simulink model "MPC_control"  (R2018a)
settings: Solver=FixedStepAuto  StartTime=0  StopTime=Tend  FixedStep=0.001  RelTol=5e-3
model workspace (MAT data in the model file):
  A_mu = 10
  B_reff = 8.386
  Cz = 7766.25
  DCT_Param : struct (value not decoded)
  D_reff = 0.25826
  Downshift_Speeds = [9.5625 12.9375 16.3125 19.6875 23.0625 26.4375 29.8125 33.1875 36.5625 39.9375 43.3125 46.6875 ... (28 elements, 4x7)]
  Pedal_Positions = [0.1 0.4 0.5 0.9]
  SUS : struct (value not decoded)
  Upshift_Speeds = [12.9375 16.3125 19.6875 33 26.4375 29.8125 33.1875 52.5 39.9375 43.3125 46.6875 77.25 ... (28 elements, 4x7)]
  VEH : struct (value not decoded)
  V_o = 16.7
  V_xlow = 1
  WH : struct (value not decoded)
  a = 1.4
  alpha_max = 1.5
  alpha_min = -1.5
  b = 1.8
  c_zo = 209651
  epsilon = 0.1
  h = 0.134
  path : struct (value not decoded)
  pio = 220000
  q_Fcx = 0
  q_Fz2 = 15.4
  q_Fzy = 0
  q_reo = 0.9974
  q_sx1 = -0.007764
  q_sx10 = 0.2824
  q_sx11 = 5.349
  q_sx12 = 0
  q_sx13 = 0
  q_sx14 = 0
  q_sx2 = 1.1915
  q_sx3 = 0.013948
  q_sx4 = 4.912
  q_sx5 = 1.02
  q_sx6 = 22.83
  q_sx7 = 0.7104
  q_sx8 = -0.023393
  q_sx9 = 0.6581
  q_sy1 = 0.00702
  q_sy2 = 0
  q_sy3 = 0.001515
  q_sy4 = 8.514e-05
  q_sy5 = 0
  q_sy6 = 0
  q_sy7 = 0.9008
  q_sy8 = -0.4089
  q_v1 = 0.0007742
  q_v2 = 0.04667
  r_Bx1 = 12.531
  r_Bx2 = 9.532
  r_Bx3 = 0
  r_By1 = 10.615
  r_By2 = 7.705
  r_By3 = 3.433e-06
  r_By4 = 0
  r_Cx1 = 1.019
  r_Cy1 = 1.0585
  r_Ex1 = -0.4487
  r_Ex2 = -0.4726
  r_Ey1 = 0.3132
  r_Ey2 = 7.63e-06
  r_Hx1 = 0.0002374
  r_Hy1 = 0.011646
  r_Hy2 = 7.63e-06
  r_Vy1 = 0.05654
  r_Vy2 = 7.63e-06
  r_Vy3 = 0
  r_Vy4 = 99.9
  r_Vy5 = 2
  r_Vy6 = 15.814
  r_o = 0.3135
  vehWidth = 2
  w = 1
symbols that are objects in the model workspace (value not decoded): VEH
undefined symbols (not defined in the file): Cok_1, Cok_2, Cok_3, Cok_4, Cok_5, Cok_6, Cok_7, Cok_8, Cok_9, Cout_1, Cout_2, Cout_3, Cout_4, Cout_5, Cout_6, Cout_7, Cout_8, Cout_9, DiscIntNeverNeededParam, Dout_1, Dout_2, Dout_3, Dout_4, Dout_5, Dout_6, Dout_7, Dout_8, Dout_9, F_1, F_2, F_3, F_4, F_5, F_6, F_7, F_8, F_9, Gd_1, Gd_2, Gd_3, Gd_4, Gd_5, Gd_6, Gd_7, Gd_8, Gd_9, Gok_1, Gok_2, Gok_3, Gok_4, Gok_5, Gok_6, Gok_7, Gok_8, Gok_9, Gsys_2, Gsys_9, Hd_1, Hd_2, Hd_3 ... (+70)
libraries: robotalgslib x10, simulink x5, sim3dlib x2, autolibutils x1, vehdynlibviscommon x1
(part 2 of 5)

== system MPC_control/Visualization/3D Engine ==
  note: 1) Add Subsystem or Model blocks as valid variant choices.
      | 2) You cannot connect blocks at this level. At simulation, connectivity is automatically
      | determined, based on the active variant and port name matching.
  VehFdbk : Inport
  3D Engine : Subsystem  VariantControl=1
  3D Engine Disabled : Subsystem  VariantControl=0

== system MPC_control/Visualization/Acceleration Cmd ==

== system MPC_control/Visualization/Brake Cmd ==

== system MPC_control/Visualization/Engine Tach [rpm] ==

== system MPC_control/Visualization/Handwheel Angle [deg] ==

== system MPC_control/Visualization/Lateral Acceleration [g] ==

== system MPC_control/Visualization/Speed [mph] ==

== system MPC_control/Visualization/Vehicle XY Plotter ==
  VehFdbk : Inport
  Bus Selector1 : BusSelector  OutputSignals=Body.phi,Body.theta,Body.psi  OutputAsBus=on
  Bus Selector2 : BusSelector  OutputSignals=Driveline.WhlAng  OutputAsBus=on
  Bus Selector3 : BusSelector  OutputSignals=Body.X,Body.Y,Body.Z  OutputAsBus=on
  Bus Selector4 : BusSelector  OutputSignals=Body.Xdot,Body.Ydot  OutputAsBus=on
  Bus to Vector{,1..3} (4 alike) : BusToVector
  Ground : Ground
  Rate Transition{1..2,5..6} (4 alike) : RateTransition  OutPortSampleTime=pltDT
  Vector Concatenate : Concatenate
  Vehicle XY Plotter : vehdynlibviscommon/Vehicle XY Plotter  bufferSize=bufferSize  w=w  a=a  b=b
  wires:
  Bus to Vector2/1 -> Rate Transition1/1  "InertCGDisp"
  Rate Transition5/1 -> Vehicle XY Plotter/1
  Bus Selector4/1 -> Bus to Vector1/1
  Rate Transition1/1 -> Vehicle XY Plotter/2
  Rate Transition6/1 -> Vehicle XY Plotter/3
  Vector Concatenate/1 -> Rate Transition6/1  "InertCGVel"
  Bus Selector1/1 -> Bus to Vector2/1
  Bus to Vector/1 -> Rate Transition5/1  "InertCGDisp"
  Bus Selector3/1 -> Bus to Vector/1
  Bus to Vector1/1 -> Vector Concatenate/1
  Ground/1 -> Vector Concatenate/2
  Bus to Vector3/1 -> Rate Transition2/1
  Bus Selector2/1 -> Bus to Vector3/1
  VehFdbk/1 -> Bus Selector1/1, Bus Selector2/1, Bus Selector4/1, Bus Selector3/1
  Rate Transition2/1 -> Vehicle XY Plotter/4

== system MPC_control/observer_of_plant/Subsystem_1 ==
  select_MPC : Inport
  select_overlap : Inport  Port=2
  select_overlap2 : Inport  Port=3
  initial : Inport  Port=4
  r(k) : Inport  Port=5
  r(k-1) : Inport  Port=6
  U(k) : Inport  Port=7
  U(k-1) : Inport  Port=8
  Y(k) : Inport  Port=9
  Demux2 : Demux  Outputs=3
  From Workspace : FromWorkspace  VariableName=flag_mod1  SampleTime=0
  gate1 : MATLAB Function  TreatAsAtomicUnit=on
  observer_of_simulator_1 : Subsystem
  simulator_1 : Subsystem
  xhat : Outport
  sye : Outport  Port=2
  ope : Outport  Port=3
  wires:
  simulator_1/2(U_overlap) -> observer_of_simulator_1/2(U_overlap)
  observer_of_simulator_1/1(xhat) -> xhat/1, simulator_1/9(xhat)
  simulator_1/1(Y_overlap) -> observer_of_simulator_1/5(Y_overlap)
  Demux2/2 -> simulator_1/4(Initial Velocities)
  Demux2/3 -> simulator_1/5(Initial HeadingAngles)
  Demux2/1 -> simulator_1/3(Initial position)
  Y(k)/1 -> observer_of_simulator_1/6(Y)
  initial/1 -> Demux2/1
  select_overlap/1 -> gate1/2(select_overlap)
  select_MPC/1 -> gate1/1(select_MPC)
  select_overlap2/1 -> gate1/3(select_overlap2)
  gate1/1(state_MPC) -> simulator_1/1(select_MPC)
  gate1/2(state_overlap) -> observer_of_simulator_1/1(select_overlap), simulator_1/2(select_overlap)
  r(k)/1 -> simulator_1/6(r(k))
  r(k-1)/1 -> observer_of_simulator_1/7(r(k-1)), simulator_1/7(r(k-1))
  U(k)/1 -> observer_of_simulator_1/3(U)
  U(k-1)/1 -> observer_of_simulator_1/4(U(k-1)), simulator_1/8(U(k-1))
  From Workspace/1 -> simulator_1/Enable
  observer_of_simulator_1/2(sye) -> sye/1
  observer_of_simulator_1/3(ope) -> ope/1

== system MPC_control/observer_of_plant/Subsystem_2 ==
  select_MPC : Inport
  select_overlap : Inport  Port=2
  select_overlap2 : Inport  Port=3
  initial : Inport  Port=4
  r(k) : Inport  Port=5
  r(k-1) : Inport  Port=6
  U(k) : Inport  Port=7
  U(k-1) : Inport  Port=8
  Y(k) : Inport  Port=9
  Demux2 : Demux  Outputs=3
  From Workspace1 : FromWorkspace  VariableName=flag_mod2  SampleTime=0
  gate2 : MATLAB Function  TreatAsAtomicUnit=on
  observer_of_simulator_2 : Subsystem
  simulator_2 : Subsystem
  xhat : Outport
  sye : Outport  Port=2
  ope : Outport  Port=3
  wires:
  simulator_2/2(U_overlap) -> observer_of_simulator_2/2(U_overlap)
  observer_of_simulator_2/1(xhat) -> xhat/1, simulator_2/9(xhat)
  simulator_2/1(Y_overlap) -> observer_of_simulator_2/5(Y_overlap)
  Demux2/2 -> simulator_2/4(Initial Velocities)
  Demux2/3 -> simulator_2/5(Initial HeadingAngles)
  Demux2/1 -> simulator_2/3(Initial position)
  Y(k)/1 -> observer_of_simulator_2/6(Y)
  initial/1 -> Demux2/1
  observer_of_simulator_2/2(sye) -> sye/1
  observer_of_simulator_2/3(ope) -> ope/1
  gate2/1(state_MPC) -> simulator_2/1(select_MPC)
  gate2/2(state_overlap) -> simulator_2/2(select_overlap), observer_of_simulator_2/1(select_overlap)
  select_MPC/1 -> gate2/1(select_MPC)
  select_overlap/1 -> gate2/2(select_overlap)
  select_overlap2/1 -> gate2/3(select_overlap2)
  From Workspace1/1 -> simulator_2/Enable
  r(k)/1 -> simulator_2/6(r(k))
  r(k-1)/1 -> observer_of_simulator_2/7(r(k-1)), simulator_2/7(r(k-1))
  U(k-1)/1 -> observer_of_simulator_2/4(U(k-1)), simulator_2/8(U(k-1))
  U(k)/1 -> observer_of_simulator_2/3(U)

== system MPC_control/observer_of_plant/Subsystem_3 ==
  select_MPC : Inport
  select_overlap : Inport  Port=2
  select_overlap2 : Inport  Port=3
  initial : Inport  Port=4
  r(k) : Inport  Port=5
  r(k-1) : Inport  Port=6
  U(k) : Inport  Port=7
  U(k-1) : Inport  Port=8
  Y(k) : Inport  Port=9
  Demux2 : Demux  Outputs=3
  From Workspace2 : FromWorkspace  VariableName=flag_mod3  SampleTime=0
  gate3 : MATLAB Function  TreatAsAtomicUnit=on
  observer_of_simulator_3 : Subsystem
  simulator_3 : Subsystem
  xhat : Outport
  sye : Outport  Port=2
  ope : Outport  Port=3
  wires:
  simulator_3/2(U_overlap) -> observer_of_simulator_3/2(U_overlap)
  simulator_3/1(Y_overlap) -> observer_of_simulator_3/5(Y_overlap)
  Demux2/2 -> simulator_3/4(Initial Velocities)
  Demux2/3 -> simulator_3/5(Initial HeadingAngles)
  Demux2/1 -> simulator_3/3(Initial position)
  Y(k)/1 -> observer_of_simulator_3/6(Y)
  initial/1 -> Demux2/1
  gate3/1(state_MPC) -> simulator_3/1(select_MPC)
  gate3/2(state_overlap) -> simulator_3/2(select_overlap), observer_of_simulator_3/1(select_overlap)
  select_MPC/1 -> gate3/1(select_MPC)
  select_overlap/1 -> gate3/2(select_overlap)
  select_overlap2/1 -> gate3/3(select_overlap2)
  r(k)/1 -> simulator_3/6(r(k))
  r(k-1)/1 -> observer_of_simulator_3/7(r(k-1)), simulator_3/7(r(k-1))
  U(k)/1 -> observer_of_simulator_3/3(U)
  U(k-1)/1 -> observer_of_simulator_3/4(U(k-1)), simulator_3/8(U(k-1))
  observer_of_simulator_3/1(xhat) -> xhat/1, simulator_3/9(xhat)
  observer_of_simulator_3/2(sye) -> sye/1
  observer_of_simulator_3/3(ope) -> ope/1
  From Workspace2/1 -> simulator_3/Enable

== system MPC_control/observer_of_plant/Subsystem_4 ==
  select_MPC : Inport
  select_overlap : Inport  Port=2
  select_overlap2 : Inport  Port=3
  initial : Inport  Port=4
  r(k) : Inport  Port=5
  r(k-1) : Inport  Port=6
  U(k) : Inport  Port=7
  U(k-1) : Inport  Port=8
  Y(k) : Inport  Port=9
  Demux2 : Demux  Outputs=3
  From Workspace3 : FromWorkspace  VariableName=flag_mod4  SampleTime=0
  gate4 : MATLAB Function  TreatAsAtomicUnit=on
  observer_of_simulator_4 : Subsystem
  simulator_4 : Subsystem
  xhat : Outport
  sye : Outport  Port=2
  ope : Outport  Port=3
  wires:
  simulator_4/2(U_overlap) -> observer_of_simulator_4/2(U_overlap)
  simulator_4/1(Y_overlap) -> observer_of_simulator_4/5(Y_overlap)
  Demux2/2 -> simulator_4/4(Initial Velocities)
  Demux2/3 -> simulator_4/5(Initial HeadingAngles)
  Demux2/1 -> simulator_4/3(Initial position)
  Y(k)/1 -> observer_of_simulator_4/6(Y)
  initial/1 -> Demux2/1
  U(k)/1 -> observer_of_simulator_4/3(U)
  gate4/1(state_MPC) -> simulator_4/1(select_MPC)
  gate4/2(state_overlap) -> simulator_4/2(select_overlap), observer_of_simulator_4/1(select_overlap)
  select_MPC/1 -> gate4/1(select_MPC)
  select_overlap/1 -> gate4/2(select_overlap)
  select_overlap2/1 -> gate4/3(select_overlap2)
  r(k)/1 -> simulator_4/6(r(k))
  r(k-1)/1 -> simulator_4/7(r(k-1)), observer_of_simulator_4/7(r(k-1))
  U(k-1)/1 -> simulator_4/8(U(k-1)), observer_of_simulator_4/4(U(k-1))
  From Workspace3/1 -> simulator_4/Enable
  observer_of_simulator_4/1(xhat) -> simulator_4/9(xhat), xhat/1
  observer_of_simulator_4/2(sye) -> sye/1
  observer_of_simulator_4/3(ope) -> ope/1

== system MPC_control/observer_of_plant/Subsystem_5 ==
  select_MPC : Inport
  select_overlap : Inport  Port=2
  select_overlap2 : Inport  Port=3
  initial : Inport  Port=4
  r(k) : Inport  Port=5
  r(k-1) : Inport  Port=6
  U(k) : Inport  Port=7
  U(k-1) : Inport  Port=8
  Y(k) : Inport  Port=9
  Demux2 : Demux  Outputs=3
  From Workspace4 : FromWorkspace  VariableName=flag_mod5  SampleTime=0
  gate5 : MATLAB Function  TreatAsAtomicUnit=on
  observer_of_simulator_5 : Subsystem
  simulator_5 : Subsystem
  xhat : Outport
  sye : Outport  Port=2
  ope : Outport  Port=3
  wires:
  simulator_5/2(U_overlap) -> observer_of_simulator_5/2(U_overlap)
  simulator_5/1(Y_overlap) -> observer_of_simulator_5/5(Y_overlap)
  Demux2/2 -> simulator_5/4(Initial Velocities)
  Demux2/3 -> simulator_5/5(Initial HeadingAngles)
  Demux2/1 -> simulator_5/3(Initial position)
  Y(k)/1 -> observer_of_simulator_5/6(Y)
  initial/1 -> Demux2/1
  gate5/1(state_MPC) -> simulator_5/1(select_MPC)
  gate5/2(state_overlap) -> observer_of_simulator_5/1(select_overlap), simulator_5/2(select_overlap)
  select_MPC/1 -> gate5/1(select_MPC)
  select_overlap/1 -> gate5/2(select_overlap)
  select_overlap2/1 -> gate5/3(select_overlap2)
  r(k)/1 -> simulator_5/6(r(k))
  U(k-1)/1 -> observer_of_simulator_5/4(U(k-1)), simulator_5/8(U(k-1))
  From Workspace4/1 -> simulator_5/Enable
  observer_of_simulator_5/1(xhat) -> simulator_5/9(xhat), xhat/1
  observer_of_simulator_5/2(sye) -> sye/1
  observer_of_simulator_5/3(ope) -> ope/1
  r(k-1)/1 -> observer_of_simulator_5/7(r(k-1)), simulator_5/7(r(k-1))
  U(k)/1 -> observer_of_simulator_5/3(U)

== system MPC_control/observer_of_plant/Subsystem_6 ==
  select_MPC : Inport
  select_overlap : Inport  Port=2
  select_overlap1 : Inport  Port=3
  initial : Inport  Port=4
  r(k) : Inport  Port=5
  r(k-1) : Inport  Port=6
  U(k) : Inport  Port=7
  U(k-1) : Inport  Port=8
  Y(k) : Inport  Port=9
  Demux2 : Demux  Outputs=3
  From Workspace5 : FromWorkspace  VariableName=flag_mod6  SampleTime=0
  gate6 : MATLAB Function  TreatAsAtomicUnit=on
  observer_of_simulator_6 : Subsystem
  simulator_6 : Subsystem
  xhat : Outport
  sye : Outport  Port=2
  ope : Outport  Port=3
  wires:
  simulator_6/2(U_overlap) -> observer_of_simulator_6/2(U_overlap)
  simulator_6/1(Y_overlap) -> observer_of_simulator_6/5(Y_overlap)
  Demux2/2 -> simulator_6/4(Initial Velocities)
  Demux2/3 -> simulator_6/5(Initial HeadingAngles)
  Demux2/1 -> simulator_6/3(Initial position)
  Y(k)/1 -> observer_of_simulator_6/6(Y)
  initial/1 -> Demux2/1
  gate6/1(state_MPC) -> simulator_6/1(select_MPC)
  gate6/2(state_overlap) -> observer_of_simulator_6/1(select_overlap), simulator_6/2(select_overlap)
  select_MPC/1 -> gate6/1(select_MPC)
  select_overlap/1 -> gate6/2(select_overlap)
  select_overlap1/1 -> gate6/3(select_overlap2)
  r(k)/1 -> simulator_6/6(r(k))
  U(k)/1 -> observer_of_simulator_6/3(U)
  U(k-1)/1 -> observer_of_simulator_6/4(U(k-1)), simulator_6/8(U(k-1))
  observer_of_simulator_6/1(xhat) -> xhat/1, simulator_6/9(xhat)
  observer_of_simulator_6/2(sye) -> sye/1
  observer_of_simulator_6/3(ope) -> ope/1
  From Workspace5/1 -> simulator_6/Enable
  r(k-1)/1 -> observer_of_simulator_6/7(r(k-1)), simulator_6/7(r(k-1))

== system MPC_control/observer_of_plant/Subsystem_7 ==
  select_MPC : Inport
  select_overlap : Inport  Port=2
  select_overlap2 : Inport  Port=3
  initial : Inport  Port=4
  r(k) : Inport  Port=5
  r(k-1) : Inport  Port=6
  U(k) : Inport  Port=7
  U(k-1) : Inport  Port=8
  Y(k) : Inport  Port=9
  Demux2 : Demux  Outputs=3
  From Workspace6 : FromWorkspace  VariableName=flag_mod7  SampleTime=0
  gate7 : MATLAB Function  TreatAsAtomicUnit=on
  observer_of_simulator_7 : Subsystem
  simulator_7 : Subsystem
  xhat : Outport
  sye : Outport  Port=2
  ope : Outport  Port=3
  wires:
  simulator_7/2(U_overlap) -> observer_of_simulator_7/2(U_overlap)
  observer_of_simulator_7/1(xhat) -> xhat/1, simulator_7/9(xhat)
  simulator_7/1(Y_overlap) -> observer_of_simulator_7/5(Y_overlap)
  Demux2/2 -> simulator_7/4(Initial Velocities)
  Demux2/3 -> simulator_7/5(Initial HeadingAngles)
  Demux2/1 -> simulator_7/3(Initial position)
  Y(k)/1 -> observer_of_simulator_7/6(Y)
  initial/1 -> Demux2/1
  gate7/1(state_MPC) -> simulator_7/1(select_MPC)
  gate7/2(state_overlap) -> simulator_7/2(select_overlap), observer_of_simulator_7/1(select_overlap)
  select_MPC/1 -> gate7/1(select_MPC)
  select_overlap/1 -> gate7/2(select_overlap)
  select_overlap2/1 -> gate7/3(select_overlap2)
  r(k)/1 -> simulator_7/6(r(k))
  r(k-1)/1 -> observer_of_simulator_7/7(r(k-1)), simulator_7/7(r(k-1))
  U(k)/1 -> observer_of_simulator_7/3(U)
  U(k-1)/1 -> observer_of_simulator_7/4(U(k-1)), simulator_7/8(U(k-1))
  observer_of_simulator_7/2(sye) -> sye/1
  observer_of_simulator_7/3(ope) -> ope/1
  From Workspace6/1 -> simulator_7/Enable

== system MPC_control/observer_of_plant/Subsystem_8 ==
  select_MPC : Inport
  select_overlap : Inport  Port=2
  select_overlap2 : Inport  Port=3
  initial : Inport  Port=4
  r(k) : Inport  Port=5
  r(k-1) : Inport  Port=6
  U(k) : Inport  Port=7
  U(k-1) : Inport  Port=8
  Y(k) : Inport  Port=9
  Demux2 : Demux  Outputs=3
  From Workspace7 : FromWorkspace  VariableName=flag_mod8  SampleTime=0
  gate8 : MATLAB Function  TreatAsAtomicUnit=on
  observer_of_simulator_8 : Subsystem
  simulator_8 : Subsystem
  xhat : Outport
  sye : Outport  Port=2
  ope : Outport  Port=3
  wires:
  simulator_8/2(U_overlap) -> observer_of_simulator_8/2(U_overlap)
  simulator_8/1(Y_overlap) -> observer_of_simulator_8/5(Y_overlap)
  Demux2/2 -> simulator_8/4(Initial Velocities)
  Demux2/3 -> simulator_8/5(Initial HeadingAngles)
  Demux2/1 -> simulator_8/3(Initial position)
  Y(k)/1 -> observer_of_simulator_8/6(Y)
  initial/1 -> Demux2/1
  gate8/1(state_MPC) -> simulator_8/1(select_MPC)
  gate8/2(state_overlap) -> observer_of_simulator_8/1(select_overlap), simulator_8/2(select_overlap)
  select_MPC/1 -> gate8/1(select_MPC)
  select_overlap/1 -> gate8/2(select_overlap)
  select_overlap2/1 -> gate8/3(select_overlap2)
  r(k)/1 -> simulator_8/6(r(k))
  r(k-1)/1 -> observer_of_simulator_8/7(r(k-1)), simulator_8/7(r(k-1))
  U(k)/1 -> observer_of_simulator_8/3(U)
  U(k-1)/1 -> observer_of_simulator_8/4(U(k-1)), simulator_8/8(U(k-1))
  observer_of_simulator_8/1(xhat) -> xhat/1, simulator_8/9(xhat)
  observer_of_simulator_8/2(sye) -> sye/1
  observer_of_simulator_8/3(ope) -> ope/1
  From Workspace7/1 -> simulator_8/Enable

== system MPC_control/observer_of_plant/Subsystem_9 ==
  select_MPC : Inport
  select_overlap : Inport  Port=2
  select_overlap2 : Inport  Port=3
  initial : Inport  Port=4
  r(k) : Inport  Port=5
  r(k-1) : Inport  Port=6
  U(k) : Inport  Port=7
  U(k-1) : Inport  Port=8
  Y(k) : Inport  Port=9
  Demux2 : Demux  Outputs=3
  From Workspace8 : FromWorkspace  VariableName=flag_mod9  SampleTime=0
  gate9 : MATLAB Function  TreatAsAtomicUnit=on
  observer_of_simulator_9 : Subsystem
  simulator_9 : Subsystem
  xhat : Outport
  sye : Outport  Port=2
  ope : Outport  Port=3
  wires:
  simulator_9/2(U_overlap) -> observer_of_simulator_9/2(U_overlap)
  observer_of_simulator_9/1(xhat) -> xhat/1, simulator_9/9(xhat)
  simulator_9/1(Y_overlap) -> observer_of_simulator_9/5(Y_overlap)
  Demux2/2 -> simulator_9/4(Initial Velocities)
  Demux2/3 -> simulator_9/5(Initial HeadingAngles)
  Demux2/1 -> simulator_9/3(Initial position)
  Y(k)/1 -> observer_of_simulator_9/6(Y)
  initial/1 -> Demux2/1
  observer_of_simulator_9/2(sye) -> sye/1
  observer_of_simulator_9/3(ope) -> ope/1
  gate9/1(state_MPC) -> simulator_9/1(select_MPC)
  gate9/2(state_overlap) -> simulator_9/2(select_overlap), observer_of_simulator_9/1(select_overlap)
  select_MPC/1 -> gate9/1(select_MPC)
  select_overlap/1 -> gate9/2(select_overlap)
  select_overlap2/1 -> gate9/3(select_overlap2)
  From Workspace8/1 -> simulator_9/Enable
  r(k)/1 -> simulator_9/6(r(k))
  r(k-1)/1 -> simulator_9/7(r(k-1)), observer_of_simulator_9/7(r(k-1))
  U(k-1)/1 -> simulator_9/8(U(k-1)), observer_of_simulator_9/4(U(k-1))
  U(k)/1 -> observer_of_simulator_9/3(U)

== system MPC_control/Controllers/Brake Controller/Brake Pressure Control ==
  note: 1) Add Subsystem or Model blocks as valid variant choices.
      | 2) You cannot connect blocks at this level. At simulation, connectivity is automatically
      | determined, based on the active variant and port name matching.
  Pref : Inport
  xdot : Inport  Port=2
  <Kappa> : Inport  Port=3
  Bang Bang ABS : Subsystem  VariantControl=1
  Open Loop : Subsystem  VariantControl=0
  PCmd : Outport

== system MPC_control/Controllers/Transmission Controller/TCM ==
  AccCmd : Inport
  EngSpd : Inport  Port=2
  VehSpdFdbk : Inport  Port=3
  function : TriggerPort  TriggerType=function-call  VariantControl=Variant
  Neutral Select : Subsystem
  Prop Shaft Speed LPF : DiscreteTransferFcn  Numerator=[0.000000000000000 0.009950166250832 ]  Denominator=[1.000000000000000 -0.990049833749168 ]  mask(DiscretizedDiscreteTransferFcn){}
      mask init:
      | %zoh
  TCM Shift Controller : Stateflow chart  TreatAsAtomicUnit=on
  prop speed to vehicle speed : Gain  Gain=0.45
  Gear Select : Outport
  wires:
  VehSpdFdbk/1 -> Prop Shaft Speed LPF/1
  TCM Shift Controller/1(GearState) -> Gear Select/1  "GearCmd"
  AccCmd/1 -> Neutral Select/1(AccCmd), TCM Shift Controller/2(pedal)  "AccCmd"
  Neutral Select/1(Neutral Select) -> TCM Shift Controller/3(Neutral)
  EngSpd/1 -> Neutral Select/2(EngSpd)
  prop speed to vehicle speed/1 -> TCM Shift Controller/1(speed)
  Prop Shaft Speed LPF/1 -> prop speed to vehicle speed/1

== system MPC_control/Visualization/3D Engine/3D Engine ==
  VehFdbk : Inport
  3D Body Offset : Constant  Value=single(0.0112)  OutDataTypeStr=single
  Add1 : Sum  Inputs=-+
  Add3 : Sum  Inputs=-+-
  Bus Selector : BusSelector  OutputSignals=Body.X,Body.Y,Body.Z,Body.phi,Body.theta,Body.psi
  Bus Selector2 : BusSelector  OutputSignals=Wheels.zAxle,Wheels.omega,Driveline.WhlAng
  Bus Selector3 : BusSelector  OutputSignals=Body.ZHP
  Constant1 : Constant  Value=zeros(4,1)  OutDataTypeStr=single
  Constant2 : Constant  Value=0  OutDataTypeStr=single
  Constant8 : Constant  Value=h
  Data Type Conversion{1,4..10,12} (9 alike) : DataTypeConversion  OutDataTypeStr=single
  Demux{,1..3} (4 alike) : Demux
  Integrator : Integrator  WrapState=on  WrappedStateUpperValue=2*pi  WrappedStateLowerValue=0  ZeroCross=off
  Part Rotation Concatenation : Subsystem
  Part Translation Concatenation : Subsystem
  Rate Transition : RateTransition  OutPortSampleTime=dt3D
  Scale : Subsystem
  Simulation 3D Engine 1 : sim3dlib/Simulation 3D Config  Priority=1  ProjectFormat=Executable  ProjectName=VehicleSimulation.exe  SceneDesc=Straight road  OpVisEn=off  Ts=dt3D
      settings: AttributesFormatString=Priority: %<Priority>
  Unary Minus : UnaryMinus
  Vehicle Actor Transform Set : sim3dlib/Simulation 3D Actor Transform Set  ActorTag=SimulinkVehicle1  ActorType=Passenger vehicle  PassVehMesh=Muscle car  VehColor=Red  NumberOfParts=5  CustNumOfParts=3  Translation=[0 0 1; 0 0 0; 0 0 0; 0 0 0; 0 0 0]  Rotation=[0 0 0; 0 0 0; 0 0 0; 0 0 0; 0 0 0]  Scale=[1 1 1; 1 1 1; 1 1 1; 1 1 1; 1 1 1]  Ts=dt3D
  wires:
  Unary Minus/1 -> Integrator/1
  Bus Selector3/1 -> Add3/2  "<ZHP>"
  Add3/1 -> Data Type Conversion12/1
  Bus Selector2/1 -> Add3/3  "<zAxle>"
  Constant8/1 -> Add3/1
  Rate Transition/1 -> Bus Selector/1, Bus Selector3/1, Bus Selector2/1
  Scale/1(ScaleOut) -> Vehicle Actor Transform Set/3
  Demux/4 -> Part Rotation Concatenation/7(WheelRearRight Ptich)
  Demux/3 -> Part Rotation Concatenation/6(WheelRearLeft Pitch)
  Demux/2 -> Part Rotation Concatenation/5(WheelFrontRight Pitch)
  Demux/1 -> Part Rotation Concatenation/4(WheelFrontLeft Pitch)
  Constant1/1 -> Demux2/1
  Bus Selector/4 -> Data Type Conversion7/1  "<phi>"
  Data Type Conversion6/1 -> Add1/1
  Part Rotation Concatenation/1(ConcatOut) -> Vehicle Actor Transform Set/2
  Part Translation Concatenation/1(ConcatOut) -> Vehicle Actor Transform Set/1
  Data Type Conversion12/1 -> Demux3/1
  Demux3/4 -> Part Translation Concatenation/15(WheelRearRightZ)
  Demux3/3 -> Part Translation Concatenation/14(WheelRearLeftZ)
  Demux3/1 -> Part Translation Concatenation/12(WheelFrontLeftZ)
  Demux3/2 -> Part Translation Concatenation/13(WheelFrontRightZ)
  VehFdbk/1 -> Rate Transition/1
  Add1/1 -> Part Translation Concatenation/3(BodyZ)
  3D Body Offset/1 -> Add1/2
  Demux1/4 -> Part Rotation Concatenation/15(WheelRearRight Yaw)
  Demux1/3 -> Part Rotation Concatenation/14(WheelRearLeft Yaw)
  Demux2/1 -> Part Rotation Concatenation/8(WheelFrontLeft Roll)
  Demux2/2 -> Part Rotation Concatenation/9(WheelFrontRight Roll)
  Demux2/3 -> Part Rotation Concatenation/10(WheelRearLeft Roll)
  Demux2/4 -> Part Rotation Concatenation/11(WheelRearRight Roll)
  Bus Selector2/3 -> Data Type Conversion9/1  "<WhlAng>"
  Bus Selector2/2 -> Unary Minus/1  "<omega>"
  Data Type Conversion9/1 -> Demux1/1
  Demux1/1 -> Part Rotation Concatenation/12(WheelFrontLeft Yaw)
  Demux1/2 -> Part Rotation Concatenation/13(WheelFrontRight Yaw)
  Integrator/1 -> Data Type Conversion1/1
  Data Type Conversion1/1 -> Demux/1
  Data Type Conversion8/1 -> Part Rotation Concatenation/2(Body Ptich)
  Data Type Conversion5/1 -> Part Translation Concatenation/2(BodyY)
  Data Type Conversion10/1 -> Part Rotation Concatenation/3(Body Yaw)
  Constant2/1 -> Part Translation Concatenation/5(WheelFrontRightX), Part Translation Concatenation/6(WheelRearLeftX), Part Translation Concatenation/7(WheelRearRightX), Part Translation Concatenation/8(WheelFrontLeftY), Part Translation Concatenation/9(WheelFrontRightY), Part Translation Concatenation/10(WheelRearLeftY), Part Translation Concatenation/11(WheelRearRightY), Part Translation Concatenation/4(WheelFrontLeftX)
  Data Type Conversion4/1 -> Part Translation Concatenation/1(BodyX)
  Data Type Conversion7/1 -> Part Rotation Concatenation/1(Body Roll)
  Bus Selector/1 -> Data Type Conversion4/1  "<X>"
  Bus Selector/2 -> Data Type Conversion5/1  "<Y>"
  Bus Selector/3 -> Data Type Conversion6/1  "<Z>"
  Bus Selector/6 -> Data Type Conversion10/1  "<psi>"
  Bus Selector/5 -> Data Type Conversion8/1  "<theta>"

== system MPC_control/Visualization/3D Engine/3D Engine Disabled ==
  VehFdbk : Inport
  Terminator : Terminator
  wires:
  VehFdbk/1 -> Terminator/1

== system MPC_control/observer_of_plant/Subsystem_1/observer_of_simulator_1 ==
  select_overlap : Inport
  U_overlap : Inport  Port=2
  U : Inport  Port=3
  U(k-1) : Inport  Port=4
  Y_overlap : Inport  Port=5
  Y : Inport  Port=6
  r(k-1) : Inport  Port=7
  Cok_1 : Gain  Gain=Cok_1  Multiplication=Matrix(K*u) (u vector)
  Cok_1* : Gain  Gain=Cok_1  Multiplication=Matrix(K*u) (u vector)
  Delay : Delay  DelayLength=1  InitialConditionSource=Input port  InitialCondition=0  ExternalReset=Rising  SampleTime=Ts
      settings: InputPortMap=u0,r5,p4
  Delay1 : Delay  DelayLength=1  InitialConditionSource=Input port  InitialCondition=0  ExternalReset=Rising  SampleTime=Ts
      settings: InputPortMap=u0,r5,p4
  Gd_1 : Gain  Gain=Gd_1  Multiplication=Matrix(K*u) (u vector)
  Gok_1 : Gain  Gain=Gok_1  Multiplication=Matrix(K*u) (u vector)
  Hd_1 : Gain  Gain=Hd_1  Multiplication=Matrix(K*u) (u vector)
  Hok_1 : Gain  Gain=Hok_1  Multiplication=Matrix(K*u) (u vector)
  Ld_1 : Gain  Gain=Ld_1  Multiplication=Matrix(K*u) (u vector)
  Ld_1* : Gain  Gain=Ld_1  Multiplication=Matrix(K*u) (u vector)
  Sum : Sum  Inputs=|-+
  Sum1 : Sum
  Sum2 : Sum  Inputs=|-+
  Sum4 : Sum  Inputs=+++
  Switch1 : Switch  Threshold=1
  Switch2 : Switch  Threshold=1
  xhat : Outport
  sye : Outport  Port=2
  ope : Outport  Port=3
  wires:
  Hd_1/1 -> Sum4/2
  Ld_1/1 -> Sum4/1
  Delay1/1 -> Hok_1/1, Hd_1/1
  U_overlap/1 -> Switch2/1
  Gd_1/1 -> Sum4/3
  Y/1 -> Sum/2, Sum2/2, Switch1/3
  U/1 -> Switch2/3
  Sum4/1 -> xhat/1, Cok_1/1, Delay/1  "xhat"
  Delay/1 -> Gok_1/1, Gd_1/1
  Y_overlap/1 -> Switch1/1
  U(k-1)/1 -> Delay1/3
  select_overlap/1 -> Delay/2, Delay1/2, Switch2/2, Switch1/2
  r(k-1)/1 -> Ld_1*/1
  Switch1/1 -> Ld_1/1
  Switch2/1 -> Delay1/1
  Ld_1*/1 -> Delay/3
  Cok_1/1 -> Sum/1
  Hok_1/1 -> Sum1/2
  Gok_1/1 -> Sum1/1
  Sum1/1 -> Cok_1*/1
  Cok_1*/1 -> Sum2/1
  Sum2/1 -> sye/1
  Sum/1 -> ope/1

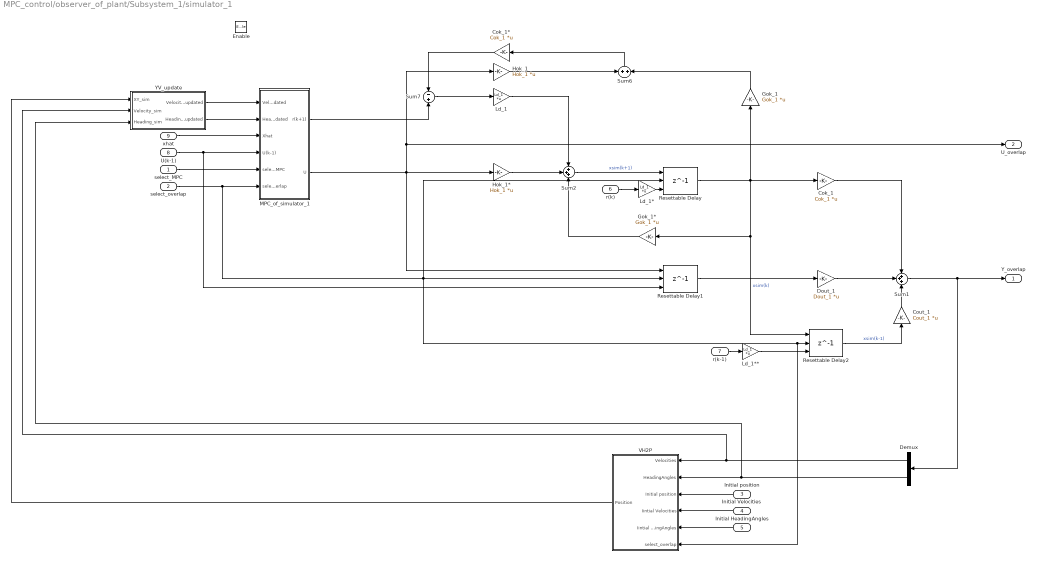
== system MPC_control/observer_of_plant/Subsystem_1/simulator_1 ==
  select_MPC : Inport
  select_overlap : Inport  Port=2
  Initial position : Inport  Port=3
  Initial Velocities : Inport  Port=4
  Initial HeadingAngles : Inport  Port=5
  r(k) : Inport  Port=6
  r(k-1) : Inport  Port=7
  U(k-1) : Inport  Port=8
  xhat : Inport  Port=9
  Enable : EnablePort
  Cok_1 : Gain  Gain=Cok_1  Multiplication=Matrix(K*u) (u vector)
  Cok_1* : Gain  Gain=Cok_1  Multiplication=Matrix(K*u) (u vector)
  Cout_1 : Gain  Gain=Cout_1  Multiplication=Matrix(K*u) (u vector)
  Demux : Demux  Outputs=2
  Dout_1 : Gain  Gain=Dout_1  Multiplication=Matrix(K*u) (u vector)
  Gok_1 : Gain  Gain=Gok_1  Multiplication=Matrix(K*u) (u vector)
  Gok_1* : Gain  Gain=Gok_1  Multiplication=Matrix(K*u) (u vector)
  Hok_1 : Gain  Gain=Hok_1  Multiplication=Matrix(K*u) (u vector)
  Hok_1* : Gain  Gain=Hok_1  Multiplication=Matrix(K*u) (u vector)
  Ld_1 : Gain  Gain=Ld_1  Multiplication=Matrix(K*u) (u vector)
  Ld_1* : Gain  Gain=Ld_1  Multiplication=Matrix(K*u) (u vector)
  Ld_1** : Gain  Gain=Ld_1  Multiplication=Matrix(K*u) (u vector)
  MPC_of_simulator_1 : Subsystem
  Resettable Delay : Delay  DelayLength=1  InitialConditionSource=Input port  ExternalReset=Rising  SampleTime=Ts
      settings: InputPortMap=u0,r5,p4
  Resettable Delay1 : Delay  DelayLength=1  InitialConditionSource=Input port  ExternalReset=Rising  SampleTime=Ts
      settings: InputPortMap=u0,r5,p4
  Resettable Delay2 : Delay  DelayLength=1  InitialConditionSource=Input port  ExternalReset=Rising  SampleTime=Ts
      settings: InputPortMap=u0,r5,p4
  Sum1 : Sum  Inputs=+++
  Sum2 : Sum  Inputs=+++
  Sum6 : Sum
  Sum7 : Sum  Inputs=-+
  VH2P : Subsystem
  YV_update : Subsystem  TreatAsAtomicUnit=on
  Y_overlap : Outport
  U_overlap : Outport  Port=2
  wires:
  Initial position/1 -> VH2P/3(Initial position)
  Sum2/1 -> Resettable Delay/1  "xsim(k+1)"
  Demux/2 -> VH2P/2(HeadingAngles), YV_update/3(Heading_sim)
  Ld_1/1 -> Sum2/1
  Sum7/1 -> Ld_1/1
  Cout_1/1 -> Sum1/3
  MPC_of_simulator_1/2(U) -> Resettable Delay1/1, Hok_1*/1, U_overlap/1, Hok_1/1
  Hok_1*/1 -> Sum2/2
  Gok_1*/1 -> Sum2/3
  Resettable Delay2/1 -> Cout_1/1  "xsim(k-1)"
  VH2P/1(Position) -> YV_update/1(XY_sim)
  Demux/1 -> YV_update/2(Velocity_sim), VH2P/1(Velocities)
  Resettable Delay/1 -> Gok_1*/1, Resettable Delay2/1, Gok_1/1, Cok_1/1  "xsim(k)"
  Hok_1/1 -> Sum6/1
  Sum1/1 -> Y_overlap/1, Demux/1
  Sum6/1 -> Cok_1*/1
  Dout_1/1 -> Sum1/2
  Resettable Delay1/1 -> Dout_1/1
  Cok_1/1 -> Sum1/1
  YV_update/2(Heading_updated) -> MPC_of_simulator_1/2(Heading_updated)
  YV_update/1(Velocity_updated) -> MPC_of_simulator_1/1(Velocity_updated)
  r(k)/1 -> Ld_1*/1
  Ld_1*/1 -> Resettable Delay/3
  U(k-1)/1 -> MPC_of_simulator_1/4(U(k-1)), Resettable Delay1/3
  r(k-1)/1 -> Ld_1**/1
  Ld_1**/1 -> Resettable Delay2/3
  Initial Velocities/1 -> VH2P/4(Iintial Velocities)
  Initial HeadingAngles/1 -> VH2P/5(Iintial HeadingAngles)
  select_overlap/1 -> MPC_of_simulator_1/6(select_overlap), Resettable Delay/2, VH2P/6(select_overlap), Resettable Delay2/2, Resettable Delay1/2
  Gok_1/1 -> Sum6/2
  Cok_1*/1 -> Sum7/1
  select_MPC/1 -> MPC_of_simulator_1/5(select_MPC)
  MPC_of_simulator_1/1(r(k+1)) -> Sum7/2
  xhat/1 -> MPC_of_simulator_1/3(Xhat)

== system MPC_control/observer_of_plant/Subsystem_2/observer_of_simulator_2 ==
  select_overlap : Inport
  U_overlap : Inport  Port=2
  U : Inport  Port=3
  U(k-1) : Inport  Port=4
  Y_overlap : Inport  Port=5
  Y : Inport  Port=6
  r(k-1) : Inport  Port=7
  Cok_2 : Gain  Gain=Cok_2  Multiplication=Matrix(K*u) (u vector)
  Cok_2* : Gain  Gain=Cok_2  Multiplication=Matrix(K*u) (u vector)
  Delay : Delay  DelayLength=1  InitialConditionSource=Input port  InitialCondition=0  ExternalReset=Rising  SampleTime=Ts
      settings: InputPortMap=u0,r5,p4
  Delay1 : Delay  DelayLength=1  InitialConditionSource=Input port  InitialCondition=0  ExternalReset=Rising  SampleTime=Ts
      settings: InputPortMap=u0,r5,p4
  Gd_2 : Gain  Gain=Gd_2  Multiplication=Matrix(K*u) (u vector)
  Gok_2 : Gain  Gain=Gok_2  Multiplication=Matrix(K*u) (u vector)
  Hd_2 : Gain  Gain=Hd_2  Multiplication=Matrix(K*u) (u vector)
  Hok_2 : Gain  Gain=Hok_2  Multiplication=Matrix(K*u) (u vector)
  Ld_2 : Gain  Gain=Ld_2  Multiplication=Matrix(K*u) (u vector)
  Ld_2* : Gain  Gain=Ld_2  Multiplication=Matrix(K*u) (u vector)
  Sum : Sum  Inputs=|-+
  Sum1 : Sum
  Sum2 : Sum  Inputs=|-+
  Sum4 : Sum  Inputs=+++
  Switch1 : Switch  Threshold=1
  Switch2 : Switch  Threshold=1
  xhat : Outport
  sye : Outport  Port=2
  ope : Outport  Port=3
  wires:
  Hd_2/1 -> Sum4/2
  Ld_2/1 -> Sum4/1
  U_overlap/1 -> Switch2/1
  Gd_2/1 -> Sum4/3
  U/1 -> Switch2/3
  Y_overlap/1 -> Switch1/1
  U(k-1)/1 -> Delay1/3
  select_overlap/1 -> Delay/2, Delay1/2, Switch2/2, Switch1/2
  r(k-1)/1 -> Ld_2*/1
  Switch1/1 -> Ld_2/1
  Switch2/1 -> Delay1/1
  Ld_2*/1 -> Delay/3
  Delay/1 -> Gok_2/1, Gd_2/1
  Sum2/1 -> sye/1
  Sum/1 -> ope/1
  Cok_2/1 -> Sum/1
  Hok_2/1 -> Sum1/2
  Delay1/1 -> Hok_2/1, Hd_2/1
  Gok_2/1 -> Sum1/1
  Y/1 -> Sum/2, Sum2/2, Switch1/3
  Cok_2*/1 -> Sum2/1
  Sum1/1 -> Cok_2*/1
  Sum4/1 -> xhat/1, Cok_2/1, Delay/1  "xhat"

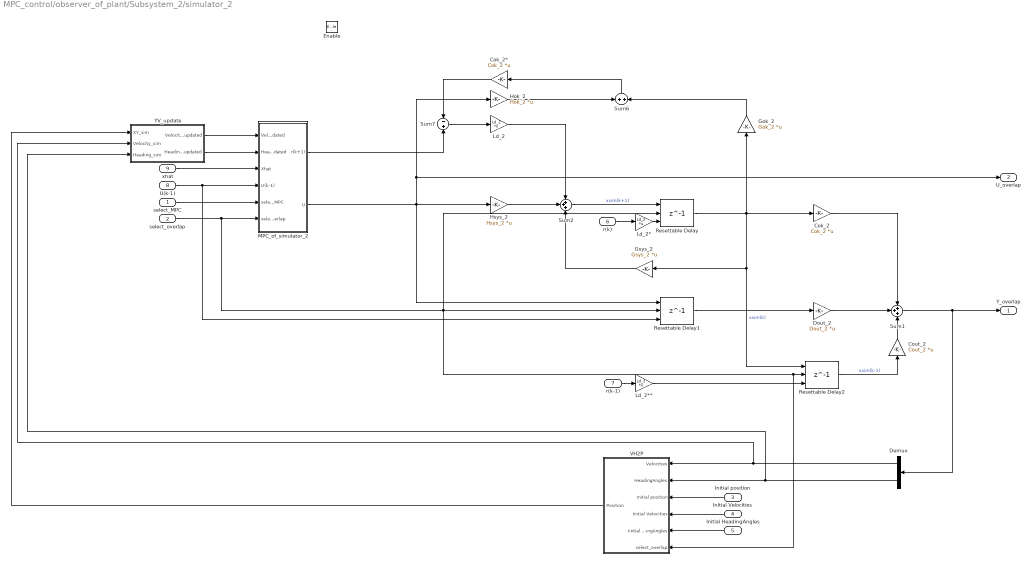
== system MPC_control/observer_of_plant/Subsystem_2/simulator_2 ==
  select_MPC : Inport
  select_overlap : Inport  Port=2
  Initial position : Inport  Port=3
  Initial Velocities : Inport  Port=4
  Initial HeadingAngles : Inport  Port=5
  r(k) : Inport  Port=6
  r(k-1) : Inport  Port=7
  U(k-1) : Inport  Port=8
  xhat : Inport  Port=9
  Enable : EnablePort
  Cok_2 : Gain  Gain=Cok_2  Multiplication=Matrix(K*u) (u vector)
  Cok_2* : Gain  Gain=Cok_2  Multiplication=Matrix(K*u) (u vector)
  Cout_2 : Gain  Gain=Cout_2  Multiplication=Matrix(K*u) (u vector)
  Demux : Demux  Outputs=2
  Dout_2 : Gain  Gain=Dout_2  Multiplication=Matrix(K*u) (u vector)
  Gok_2 : Gain  Gain=Gok_2  Multiplication=Matrix(K*u) (u vector)
  Gsys_2 : Gain  Gain=Gsys_2  Multiplication=Matrix(K*u) (u vector)
  Hok_2 : Gain  Gain=Hok_2  Multiplication=Matrix(K*u) (u vector)
  Hsys_2 : Gain  Gain=Hsys_2  Multiplication=Matrix(K*u) (u vector)
  Ld_2 : Gain  Gain=Ld_2  Multiplication=Matrix(K*u) (u vector)
  Ld_2* : Gain  Gain=Ld_2  Multiplication=Matrix(K*u) (u vector)
  Ld_2** : Gain  Gain=Ld_2  Multiplication=Matrix(K*u) (u vector)
  MPC_of_simulator_2 : Subsystem
  Resettable Delay : Delay  DelayLength=1  InitialConditionSource=Input port  ExternalReset=Rising  SampleTime=Ts
      settings: InputPortMap=u0,r5,p4
  Resettable Delay1 : Delay  DelayLength=1  InitialConditionSource=Input port  ExternalReset=Rising  SampleTime=Ts
      settings: InputPortMap=u0,r5,p4
  Resettable Delay2 : Delay  DelayLength=1  InitialConditionSource=Input port  ExternalReset=Rising  SampleTime=Ts
      settings: InputPortMap=u0,r5,p4
  Sum1 : Sum  Inputs=+++
  Sum2 : Sum  Inputs=+++
  Sum6 : Sum
  Sum7 : Sum  Inputs=-+
  VH2P : Subsystem
  YV_update : Subsystem  TreatAsAtomicUnit=on
  Y_overlap : Outport
  U_overlap : Outport  Port=2
  wires:
  Initial position/1 -> VH2P/3(Initial position)
  Sum2/1 -> Resettable Delay/1  "xsim(k+1)"
  Demux/2 -> VH2P/2(HeadingAngles), YV_update/3(Heading_sim)
  Ld_2/1 -> Sum2/1
  Sum7/1 -> Ld_2/1
  Cout_2/1 -> Sum1/3
  MPC_of_simulator_2/2(U) -> Hok_2/1, U_overlap/1, Resettable Delay1/1, Hsys_2/1
  Hsys_2/1 -> Sum2/2
  Gsys_2/1 -> Sum2/3
  Resettable Delay2/1 -> Cout_2/1  "xsim(k-1)"
  VH2P/1(Position) -> YV_update/1(XY_sim)
  Demux/1 -> YV_update/2(Velocity_sim), VH2P/1(Velocities)
  Resettable Delay/1 -> Gsys_2/1, Resettable Delay2/1, Gok_2/1, Cok_2/1  "xsim(k)"
  Hok_2/1 -> Sum6/1
  Sum6/1 -> Cok_2*/1
  Dout_2/1 -> Sum1/2
  Resettable Delay1/1 -> Dout_2/1
  Cok_2/1 -> Sum1/1
  YV_update/2(Heading_updated) -> MPC_of_simulator_2/2(Heading_updated)
  xhat/1 -> MPC_of_simulator_2/3(Xhat)
  YV_update/1(Velocity_updated) -> MPC_of_simulator_2/1(Velocity_updated)
  r(k)/1 -> Ld_2*/1
  Ld_2*/1 -> Resettable Delay/3
  U(k-1)/1 -> MPC_of_simulator_2/4(U(k-1)), Resettable Delay1/3
  r(k-1)/1 -> Ld_2**/1
  Ld_2**/1 -> Resettable Delay2/3
  Initial Velocities/1 -> VH2P/4(Iintial Velocities)
  Initial HeadingAngles/1 -> VH2P/5(Iintial HeadingAngles)
  select_overlap/1 -> MPC_of_simulator_2/6(select_overlap), Resettable Delay/2, VH2P/6(select_overlap), Resettable Delay2/2, Resettable Delay1/2
  Gok_2/1 -> Sum6/2
  Cok_2*/1 -> Sum7/1
  select_MPC/1 -> MPC_of_simulator_2/5(select_MPC)
  Sum1/1 -> Demux/1, Y_overlap/1
  MPC_of_simulator_2/1(r(k+1)) -> Sum7/2

== system MPC_control/observer_of_plant/Subsystem_3/observer_of_simulator_3 ==
  select_overlap : Inport
  U_overlap : Inport  Port=2
  U : Inport  Port=3
  U(k-1) : Inport  Port=4
  Y_overlap : Inport  Port=5
  Y : Inport  Port=6
  r(k-1) : Inport  Port=7
  Cok_3 : Gain  Gain=Cok_3  Multiplication=Matrix(K*u) (u vector)
  Cok_3* : Gain  Gain=Cok_3  Multiplication=Matrix(K*u) (u vector)
  Delay : Delay  DelayLength=1  InitialConditionSource=Input port  InitialCondition=0  ExternalReset=Rising  SampleTime=Ts
      settings: InputPortMap=u0,r5,p4
  Delay1 : Delay  DelayLength=1  InitialConditionSource=Input port  InitialCondition=0  ExternalReset=Rising  SampleTime=Ts
      settings: InputPortMap=u0,r5,p4
  Gd_3 : Gain  Gain=Gd_3  Multiplication=Matrix(K*u) (u vector)
  Gok_3 : Gain  Gain=Gok_3  Multiplication=Matrix(K*u) (u vector)
  Hd_3 : Gain  Gain=Hd_3  Multiplication=Matrix(K*u) (u vector)
  Hok_3 : Gain  Gain=Hok_3  Multiplication=Matrix(K*u) (u vector)
  Ld_3 : Gain  Gain=Ld_3  Multiplication=Matrix(K*u) (u vector)
  Ld_3* : Gain  Gain=Ld_3  Multiplication=Matrix(K*u) (u vector)
  Sum : Sum  Inputs=|-+
  Sum1 : Sum
  Sum2 : Sum  Inputs=|-+
  Sum4 : Sum  Inputs=+++
  Switch1 : Switch  Threshold=1
  Switch2 : Switch  Threshold=1
  xhat : Outport
  sye : Outport  Port=2
  ope : Outport  Port=3
  wires:
  Hd_3/1 -> Sum4/2
  Ld_3/1 -> Sum4/1
  U_overlap/1 -> Switch2/1
  Gd_3/1 -> Sum4/3
  U/1 -> Switch2/3
  Y_overlap/1 -> Switch1/1
  U(k-1)/1 -> Delay1/3
  select_overlap/1 -> Delay/2, Delay1/2, Switch2/2, Switch1/2
  r(k-1)/1 -> Ld_3*/1
  Switch1/1 -> Ld_3/1
  Switch2/1 -> Delay1/1
  Ld_3*/1 -> Delay/3
  Delay/1 -> Gok_3/1, Gd_3/1
  Sum2/1 -> sye/1
  Sum/1 -> ope/1
  Cok_3/1 -> Sum/1
  Hok_3/1 -> Sum1/2
  Delay1/1 -> Hok_3/1, Hd_3/1
  Gok_3/1 -> Sum1/1
  Y/1 -> Sum/2, Sum2/2, Switch1/3
  Cok_3*/1 -> Sum2/1
  Sum1/1 -> Cok_3*/1
  Sum4/1 -> xhat/1, Cok_3/1, Delay/1  "xhat"

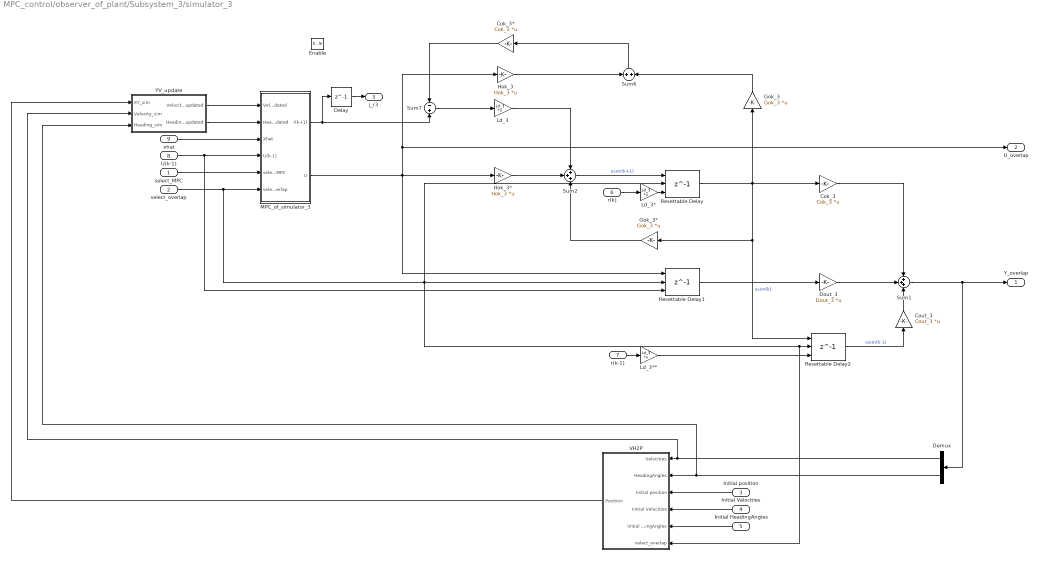
== system MPC_control/observer_of_plant/Subsystem_3/simulator_3 ==
  select_MPC : Inport
  select_overlap : Inport  Port=2
  Initial position : Inport  Port=3
  Initial Velocities : Inport  Port=4
  Initial HeadingAngles : Inport  Port=5
  r(k) : Inport  Port=6
  r(k-1) : Inport  Port=7
  U(k-1) : Inport  Port=8
  xhat : Inport  Port=9
  Enable : EnablePort
  Cok_3 : Gain  Gain=Cok_3  Multiplication=Matrix(K*u) (u vector)
  Cok_3* : Gain  Gain=Cok_3  Multiplication=Matrix(K*u) (u vector)
  Cout_3 : Gain  Gain=Cout_3  Multiplication=Matrix(K*u) (u vector)
  Delay : Delay  DelayLength=1  SampleTime=Ts
  Demux : Demux  Outputs=2
  Dout_3 : Gain  Gain=Dout_3  Multiplication=Matrix(K*u) (u vector)
  Gok_3 : Gain  Gain=Gok_3  Multiplication=Matrix(K*u) (u vector)
  Gok_3* : Gain  Gain=Gok_3  Multiplication=Matrix(K*u) (u vector)
  Hok_3 : Gain  Gain=Hok_3  Multiplication=Matrix(K*u) (u vector)
  Hok_3* : Gain  Gain=Hok_3  Multiplication=Matrix(K*u) (u vector)
  Ld_3 : Gain  Gain=Ld_3  Multiplication=Matrix(K*u) (u vector)
  Ld_3* : Gain  Gain=Ld_3  Multiplication=Matrix(K*u) (u vector)
  Ld_3** : Gain  Gain=Ld_3  Multiplication=Matrix(K*u) (u vector)
  MPC_of_simulator_3 : Subsystem
  Resettable Delay : Delay  DelayLength=1  InitialConditionSource=Input port  ExternalReset=Rising  SampleTime=Ts
      settings: InputPortMap=u0,r5,p4
  Resettable Delay1 : Delay  DelayLength=1  InitialConditionSource=Input port  ExternalReset=Rising  SampleTime=Ts
      settings: InputPortMap=u0,r5,p4
  Resettable Delay2 : Delay  DelayLength=1  InitialConditionSource=Input port  ExternalReset=Rising  SampleTime=Ts
      settings: InputPortMap=u0,r5,p4
  Sum1 : Sum  Inputs=+++
  Sum2 : Sum  Inputs=+++
  Sum6 : Sum
  Sum7 : Sum  Inputs=-+
  VH2P : Subsystem
  YV_update : Subsystem  TreatAsAtomicUnit=on
  Y_overlap : Outport
  U_overlap : Outport  Port=2
  j_r3 : Outport  Port=3
  wires:
  Sum2/1 -> Resettable Delay/1  "xsim(k+1)"
  Demux/2 -> VH2P/2(HeadingAngles), YV_update/3(Heading_sim)
  Ld_3/1 -> Sum2/1
  Sum7/1 -> Ld_3/1
  Cout_3/1 -> Sum1/3
  MPC_of_simulator_3/2(U) -> Resettable Delay1/1, Hok_3*/1, U_overlap/1, Hok_3/1
  Hok_3*/1 -> Sum2/2
  Gok_3*/1 -> Sum2/3
  Resettable Delay2/1 -> Cout_3/1  "xsim(k-1)"
  VH2P/1(Position) -> YV_update/1(XY_sim)
  Demux/1 -> YV_update/2(Velocity_sim), VH2P/1(Velocities)
  Resettable Delay/1 -> Gok_3*/1, Resettable Delay2/1, Gok_3/1, Cok_3/1  "xsim(k)"
  Hok_3/1 -> Sum6/1
  Sum6/1 -> Cok_3*/1
  Dout_3/1 -> Sum1/2
  Resettable Delay1/1 -> Dout_3/1
  Cok_3/1 -> Sum1/1
  YV_update/2(Heading_updated) -> MPC_of_simulator_3/2(Heading_updated)
  YV_update/1(Velocity_updated) -> MPC_of_simulator_3/1(Velocity_updated)
  r(k)/1 -> Ld_3*/1
  Ld_3*/1 -> Resettable Delay/3
  U(k-1)/1 -> MPC_of_simulator_3/4(U(k-1)), Resettable Delay1/3
  r(k-1)/1 -> Ld_3**/1
  Ld_3**/1 -> Resettable Delay2/3
  select_overlap/1 -> MPC_of_simulator_3/6(select_overlap), Resettable Delay/2, VH2P/6(select_overlap), Resettable Delay2/2, Resettable Delay1/2
  Gok_3/1 -> Sum6/2
  Cok_3*/1 -> Sum7/1
  select_MPC/1 -> MPC_of_simulator_3/5(select_MPC)
  Sum1/1 -> Demux/1, Y_overlap/1
  Delay/1 -> j_r3/1
  MPC_of_simulator_3/1(r(k+1)) -> Delay/1, Sum7/2
  Initial position/1 -> VH2P/3(Initial position)
  Initial Velocities/1 -> VH2P/4(Iintial Velocities)
  Initial HeadingAngles/1 -> VH2P/5(Iintial HeadingAngles)
  xhat/1 -> MPC_of_simulator_3/3(Xhat)

== system MPC_control/observer_of_plant/Subsystem_4/observer_of_simulator_4 ==
  select_overlap : Inport
  U_overlap : Inport  Port=2
  U : Inport  Port=3
  U(k-1) : Inport  Port=4
  Y_overlap : Inport  Port=5
  Y : Inport  Port=6
  r(k-1) : Inport  Port=7
  Cok_4 : Gain  Gain=Cok_4  Multiplication=Matrix(K*u) (u vector)
  Cok_4* : Gain  Gain=Cok_4  Multiplication=Matrix(K*u) (u vector)
  Delay : Delay  DelayLength=1  InitialConditionSource=Input port  InitialCondition=0  ExternalReset=Rising  SampleTime=Ts
      settings: InputPortMap=u0,r5,p4
  Delay1 : Delay  DelayLength=1  InitialConditionSource=Input port  InitialCondition=0  ExternalReset=Rising  SampleTime=Ts
      settings: InputPortMap=u0,r5,p4
  Gd_4 : Gain  Gain=Gd_4  Multiplication=Matrix(K*u) (u vector)
  Gok_4 : Gain  Gain=Gok_4  Multiplication=Matrix(K*u) (u vector)
  Hd_4 : Gain  Gain=Hd_4  Multiplication=Matrix(K*u) (u vector)
  Hok_4 : Gain  Gain=Hok_4  Multiplication=Matrix(K*u) (u vector)
  Ld_4 : Gain  Gain=Ld_4  Multiplication=Matrix(K*u) (u vector)
  Ld_4* : Gain  Gain=Ld_4  Multiplication=Matrix(K*u) (u vector)
  Sum : Sum  Inputs=|-+
  Sum1 : Sum
  Sum2 : Sum  Inputs=|-+
  Sum4 : Sum  Inputs=+++
  Switch1 : Switch  Threshold=1
  Switch2 : Switch  Threshold=1
  xhat : Outport
  sye : Outport  Port=2
  ope : Outport  Port=3
  wires:
  Hd_4/1 -> Sum4/2
  Ld_4/1 -> Sum4/1
  U_overlap/1 -> Switch2/1
  Gd_4/1 -> Sum4/3
  U/1 -> Switch2/3
  Y_overlap/1 -> Switch1/1
  U(k-1)/1 -> Delay1/3
  select_overlap/1 -> Delay/2, Delay1/2, Switch2/2, Switch1/2
  r(k-1)/1 -> Ld_4*/1
  Switch1/1 -> Ld_4/1
  Switch2/1 -> Delay1/1
  Ld_4*/1 -> Delay/3
  Delay/1 -> Gok_4/1, Gd_4/1
  Sum2/1 -> sye/1
  Sum/1 -> ope/1
  Cok_4/1 -> Sum/1
  Hok_4/1 -> Sum1/2
  Delay1/1 -> Hok_4/1, Hd_4/1
  Gok_4/1 -> Sum1/1
  Y/1 -> Sum/2, Sum2/2, Switch1/3
  Cok_4*/1 -> Sum2/1
  Sum1/1 -> Cok_4*/1
  Sum4/1 -> xhat/1, Cok_4/1, Delay/1  "xhat"

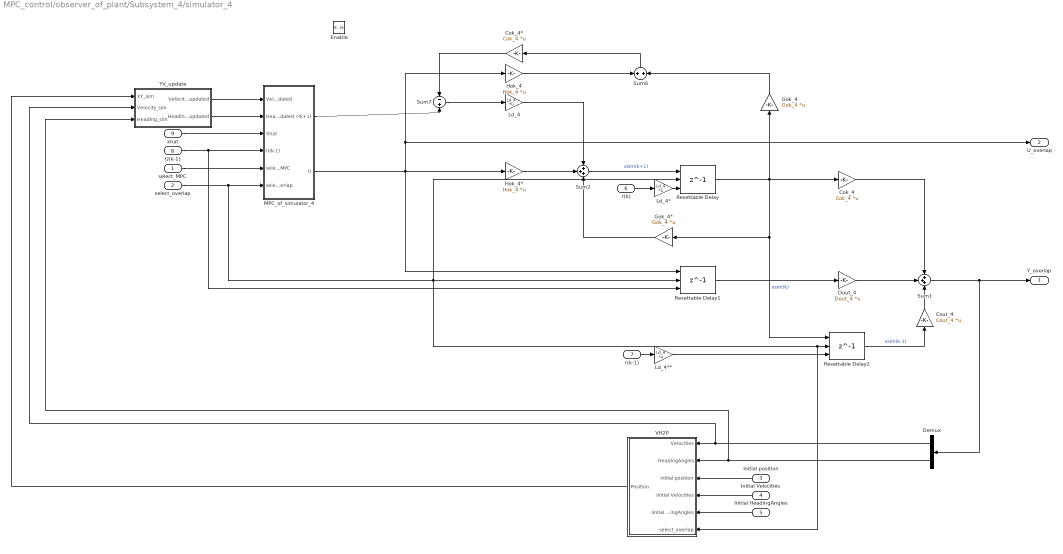
== system MPC_control/observer_of_plant/Subsystem_4/simulator_4 ==
  select_MPC : Inport
  select_overlap : Inport  Port=2
  Initial position : Inport  Port=3
  Initial Velocities : Inport  Port=4
  Initial HeadingAngles : Inport  Port=5
  r(k) : Inport  Port=6
  r(k-1) : Inport  Port=7
  U(k-1) : Inport  Port=8
  xhat : Inport  Port=9
  Enable : EnablePort
  Cok_4 : Gain  Gain=Cok_4  Multiplication=Matrix(K*u) (u vector)
  Cok_4* : Gain  Gain=Cok_4  Multiplication=Matrix(K*u) (u vector)
  Cout_4 : Gain  Gain=Cout_4  Multiplication=Matrix(K*u) (u vector)
  Demux : Demux  Outputs=2
  Dout_4 : Gain  Gain=Dout_4  Multiplication=Matrix(K*u) (u vector)
  Gok_4 : Gain  Gain=Gok_4  Multiplication=Matrix(K*u) (u vector)
  Gok_4* : Gain  Gain=Gok_4  Multiplication=Matrix(K*u) (u vector)
  Hok_4 : Gain  Gain=Hok_4  Multiplication=Matrix(K*u) (u vector)
  Hok_4* : Gain  Gain=Hok_4  Multiplication=Matrix(K*u) (u vector)
  Ld_4 : Gain  Gain=Ld_4  Multiplication=Matrix(K*u) (u vector)
  Ld_4* : Gain  Gain=Ld_4  Multiplication=Matrix(K*u) (u vector)
  Ld_4** : Gain  Gain=Ld_4  Multiplication=Matrix(K*u) (u vector)
  MPC_of_simulator_4 : Subsystem
  Resettable Delay : Delay  DelayLength=1  InitialConditionSource=Input port  ExternalReset=Rising  SampleTime=Ts
      settings: InputPortMap=u0,r5,p4
  Resettable Delay1 : Delay  DelayLength=1  InitialConditionSource=Input port  ExternalReset=Rising  SampleTime=Ts
      settings: InputPortMap=u0,r5,p4
  Resettable Delay2 : Delay  DelayLength=1  InitialConditionSource=Input port  ExternalReset=Rising  SampleTime=Ts
      settings: InputPortMap=u0,r5,p4
  Sum1 : Sum  Inputs=+++
  Sum2 : Sum  Inputs=+++
  Sum6 : Sum
  Sum7 : Sum  Inputs=-+
  VH2P : Subsystem
  YV_update : Subsystem  TreatAsAtomicUnit=on
  Y_overlap : Outport
  U_overlap : Outport  Port=2
  wires:
  Initial position/1 -> VH2P/3(Initial position)
  Sum2/1 -> Resettable Delay/1  "xsim(k+1)"
  Demux/2 -> VH2P/2(HeadingAngles), YV_update/3(Heading_sim)
  Ld_4/1 -> Sum2/1
  Sum7/1 -> Ld_4/1
  Cout_4/1 -> Sum1/3
  Hok_4*/1 -> Sum2/2
  Gok_4*/1 -> Sum2/3
  Resettable Delay2/1 -> Cout_4/1  "xsim(k-1)"
  VH2P/1(Position) -> YV_update/1(XY_sim)
  Demux/1 -> YV_update/2(Velocity_sim), VH2P/1(Velocities)
  Resettable Delay/1 -> Gok_4*/1, Resettable Delay2/1, Gok_4/1, Cok_4/1  "xsim(k)"
  Hok_4/1 -> Sum6/1
  Sum6/1 -> Cok_4*/1
  Dout_4/1 -> Sum1/2
  Resettable Delay1/1 -> Dout_4/1
  Cok_4/1 -> Sum1/1
  YV_update/2(Heading_updated) -> MPC_of_simulator_4/2(Heading_updated)
  YV_update/1(Velocity_updated) -> MPC_of_simulator_4/1(Velocity_updated)
  r(k)/1 -> Ld_4*/1
  Ld_4*/1 -> Resettable Delay/3
  U(k-1)/1 -> MPC_of_simulator_4/4(U(k-1)), Resettable Delay1/3
  r(k-1)/1 -> Ld_4**/1
  Ld_4**/1 -> Resettable Delay2/3
  Initial Velocities/1 -> VH2P/4(Iintial Velocities)
  Initial HeadingAngles/1 -> VH2P/5(Iintial HeadingAngles)
  select_overlap/1 -> MPC_of_simulator_4/6(select_overlap), Resettable Delay/2, VH2P/6(select_overlap), Resettable Delay2/2, Resettable Delay1/2
  Gok_4/1 -> Sum6/2
  Cok_4*/1 -> Sum7/1
  select_MPC/1 -> MPC_of_simulator_4/5(select_MPC)
  Sum1/1 -> Y_overlap/1, Demux/1
  MPC_of_simulator_4/1(r(k+1)) -> Sum7/2
  MPC_of_simulator_4/2(U) -> Hok_4*/1, Hok_4/1, U_overlap/1, Resettable Delay1/1
  xhat/1 -> MPC_of_simulator_4/3(Xhat)

== system MPC_control/observer_of_plant/Subsystem_5/observer_of_simulator_5 ==
  select_overlap : Inport
  U_overlap : Inport  Port=2
  U : Inport  Port=3
  U(k-1) : Inport  Port=4
  Y_overlap : Inport  Port=5
  Y : Inport  Port=6
  r(k-1) : Inport  Port=7
  Cok_5 : Gain  Gain=Cok_5  Multiplication=Matrix(K*u) (u vector)
  Cok_5* : Gain  Gain=Cok_5  Multiplication=Matrix(K*u) (u vector)
  Delay : Delay  DelayLength=1  InitialConditionSource=Input port  InitialCondition=0  ExternalReset=Rising  SampleTime=Ts
      settings: InputPortMap=u0,r5,p4
  Delay1 : Delay  DelayLength=1  InitialConditionSource=Input port  InitialCondition=0  ExternalReset=Rising  SampleTime=Ts
      settings: InputPortMap=u0,r5,p4
  Gd_5 : Gain  Gain=Gd_5  Multiplication=Matrix(K*u) (u vector)
  Gok_5 : Gain  Gain=Gok_5  Multiplication=Matrix(K*u) (u vector)
  Hd_5 : Gain  Gain=Hd_5  Multiplication=Matrix(K*u) (u vector)
  Hok_5 : Gain  Gain=Hok_5  Multiplication=Matrix(K*u) (u vector)
  Ld_5 : Gain  Gain=Ld_5  Multiplication=Matrix(K*u) (u vector)
  Ld_5* : Gain  Gain=Ld_5  Multiplication=Matrix(K*u) (u vector)
  Sum : Sum  Inputs=|-+
  Sum1 : Sum
  Sum2 : Sum  Inputs=|-+
  Sum4 : Sum  Inputs=+++
  Switch1 : Switch  Threshold=1
  Switch2 : Switch  Threshold=1
  xhat : Outport
  sye : Outport  Port=2
  ope : Outport  Port=3
  wires:
  Hd_5/1 -> Sum4/2
  Ld_5/1 -> Sum4/1
  U_overlap/1 -> Switch2/1
  Gd_5/1 -> Sum4/3
  U/1 -> Switch2/3
  Y_overlap/1 -> Switch1/1
  U(k-1)/1 -> Delay1/3
  select_overlap/1 -> Delay/2, Delay1/2, Switch2/2, Switch1/2
  r(k-1)/1 -> Ld_5*/1
  Switch1/1 -> Ld_5/1
  Switch2/1 -> Delay1/1
  Ld_5*/1 -> Delay/3
  Delay/1 -> Gok_5/1, Gd_5/1
  Sum2/1 -> sye/1
  Sum/1 -> ope/1
  Cok_5/1 -> Sum/1
  Hok_5/1 -> Sum1/2
  Delay1/1 -> Hok_5/1, Hd_5/1
  Gok_5/1 -> Sum1/1
  Y/1 -> Sum/2, Sum2/2, Switch1/3
  Cok_5*/1 -> Sum2/1
  Sum1/1 -> Cok_5*/1
  Sum4/1 -> xhat/1, Cok_5/1, Delay/1  "xhat"
